simulink model "simulationIntegrationEquationSolver"  (R2022a)
settings: Solver=VariableStepAuto  StartTime=0.0  StopTime=10.0  RelTol=1e-3
settings Model: Creator=Waleed  LastModifiedBy=Waleed

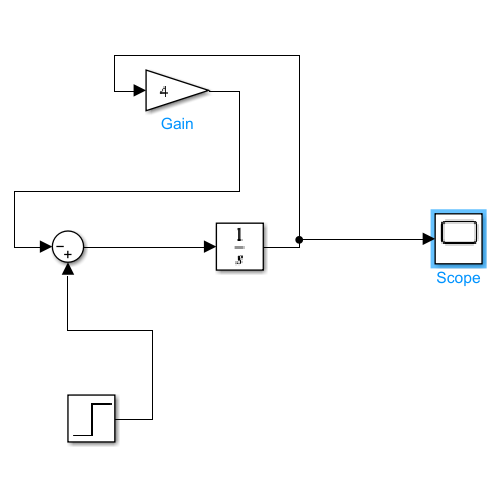
[thumbnail: Simulink's stored preview of the top-level diagram]
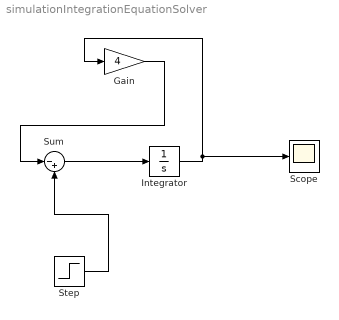
== system simulationIntegrationEquationSolver ==
  Gain : Gain  Gain=4
  Integrator : Integrator
  Scope : Scope
  Step : Step  SampleTime=0
  Sum : Sum  Inputs=|-+
  wires:
  Step/1 -> Sum/2
  Sum/1 -> Integrator/1
  Integrator/1 -> Scope/1, Gain/1
  Gain/1 -> Sum/1
